simulink model "glucose_minimal_model"  (R2014a)
settings: Solver=ode3  StartTime=0.0  StopTime=300  FixedStep=0.01  RelTol=1e-3
values from neighbouring files (symbols this model uses):
  G0 = Gb + p0    (= 276)    [Modified_Bergman.m]    (also in data.m = 287)
  Gb = 81    [Modified_Bergman.m]    (also in data.m = 92)
  Ib = 15    [Modified_Bergman.m]    (also in data.m = 7.3)
  p1 = 0.028735    [Modified_Bergman.m]    (also in data.m = 0.03082)
  p2 = 0.028344    [Modified_Bergman.m]    (also in data.m = 0.02093)
  p3 = 5.035E-5    (= 5.035e-05)    [Modified_Bergman.m]    (also in data.m = 1.06e-05)
  X0 = 0    [Modified_Bergman.m]    (also in data.m)
settings Model: Creator=sameer  LastModifiedBy=sameer

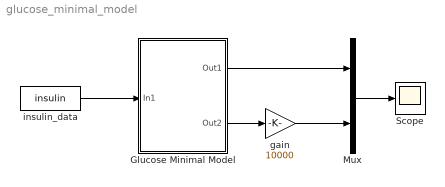
== system glucose_minimal_model ==
  Glucose Minimal Model : Subsystem
  Mux : Mux  Inputs=2
  Scope : Scope
      settings: SaveName=X1
  gain : Gain  Gain=10000
  "insulin_data " : FromWorkspace  VariableName=insulin  SampleTime=0.01
  wires:
  "insulin_data "/1 -> Glucose Minimal Model/1(In1)
  Glucose Minimal Model/1(Out1) -> Mux/1
  Glucose Minimal Model/2(Out2) -> gain/1
  Mux/1 -> Scope/1
  gain/1 -> Mux/2

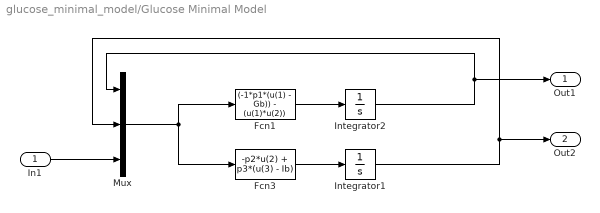
== system glucose_minimal_model/Glucose Minimal Model ==
  In1 : Inport
  Fcn1 : Fcn  Expr=(-1*p1*(u(1) - Gb)) - (u(1)*u(2))
  Fcn3 : Fcn  Expr=-p2*u(2) + p3*(u(3) - Ib)
  Integrator1 : Integrator  InitialCondition=X0
  Integrator2 : Integrator  InitialCondition=G0
  Mux : Mux  Inputs=3
  Out1 : Outport
  Out2 : Outport  Port=2
  wires:
  Mux/1 -> Fcn3/1, Fcn1/1
  Integrator2/1 -> Mux/1, Out1/1
  Fcn3/1 -> Integrator1/1
  Fcn1/1 -> Integrator2/1
  Integrator1/1 -> Mux/2, Out2/1
  In1/1 -> Mux/3
